simulink model "LPC_rec"  (Simulink 5.0)
settings: Solver=FixedStepDiscrete  SolverMode=SingleTasking  StartTime=0.0  StopTime=inf  RelTol=1e-3
PreLoadFcn:
  | load mtlb;
libraries: dspstat3 x2, dspbuff3 x2, dspsigops x2, dspsolvers x2, dsparch4 x2, dspsrcs4 x2
settings Model: RequirementInfo=9  CovMetricSettings=d  Creator=dshpak  LastModifiedBy=Miky  ExtModeTrigMode=oneshot  ExtModeArmWhenConnect=off  ExtModeAutoUpdateStatusClock=off  SaveTime=off  SaveOutput=off  SaveFormat=Structure  LimitDataPoints=off  IntegerOverflowMsg=none  BlockReductionOpt=off  BooleanDataType=off  RTWOptions="-aEnforceIntegerDowncast=1 -aExtMode=0 -aExtModeTesting=0 -aFoldNonRolledExpr=1 -aForceParamTrailComments=0 -aGenerateComments=1 -aGenerateReport=0 -aIgnoreCustomStorageClasses=1 -aIncDataTypeInIds=0 -aIncHierarchyInIds=0 -aInlineInvariantSignals=0 -aInlinedPrmAccess=\"Literals\" -aLocalBlockOutputs=1 -aLogVarNameModifier=\"rt_\" -aMaxRTWIdLen=31 -aPrefixModelToSubsysFcnNames=1 -aRTWVerbose=1 -aRollThreshold=5 -aShowEliminatedStatements=1"

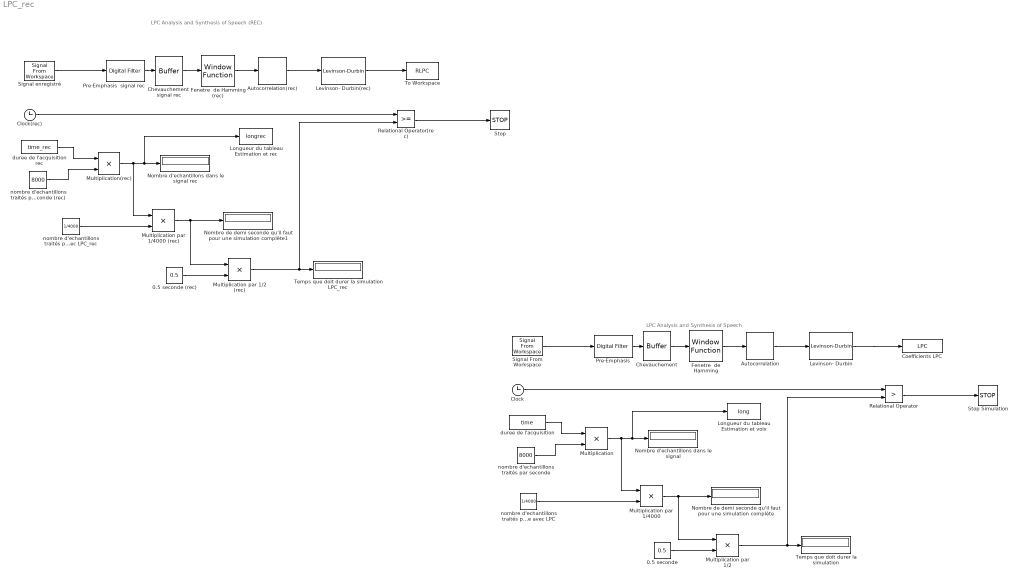
== system LPC_rec ==
  note: LPC Analysis and Synthesis of Speech
  note: LPC Analysis and Synthesis of Speech
      | (REC)
  0.5 seconde : Constant  Value=0.5
  0.5 seconde (rec) : Constant  Value=0.5
  Autocorrelation : dspstat3/Autocorrelation  AllPositiveLags=off  maxlag=12  bias=Biased  domain=Time
  Autocorrelation(rec) : dspstat3/Autocorrelation  AllPositiveLags=off  maxlag=12  bias=Biased  domain=Time
  Chevauchement : dspbuff3/Buffer  N=160  V=80  ic=0
  Chevauchement  signal rec : dspbuff3/Buffer  N=160  V=80  ic=0
  Clock : Clock
      settings: Decimation=10
  Clock(rec) : Clock
      settings: Decimation=10
  Coefficients LPC : ToWorkspace  VariableName=LPC  SampleTime=-1  SaveFormat=Array
  Fenetre  de Hamming : dspsigops/Window Function  winmode=Apply window to input  wintype=Hamming  N=64  Rs=50  beta=10  winsamp=Symmetric  UserWindow=hamming  OptParams=off  UserParams={1.0}  datatype=Double
  Fenetre  de Hamming (rec) : dspsigops/Window Function  winmode=Apply window to input  wintype=Hamming  N=64  Rs=50  beta=10  winsamp=Symmetric  UserWindow=hamming  OptParams=off  UserParams={1.0}  datatype=Double
  Levinson- Durbin : dspsolvers/Levinson-Durbin  coeffOutFcn=A  outP=off  zeroInpHandling=on
  Levinson- Durbin(rec) : dspsolvers/Levinson-Durbin  coeffOutFcn=A  outP=off  zeroInpHandling=on
  Longueur du tableau Estimation et rec : ToWorkspace  VariableName=longrec  SampleTime=-1  SaveFormat=StructureWithTime
      settings: MaxDataPoints=1
  Longueur du tableau Estimation et voix : ToWorkspace  VariableName=long  SampleTime=-1  SaveFormat=StructureWithTime
      settings: MaxDataPoints=1
  Multiplication : Product  Inputs=**  ShowAdditionalParam=on  OutDataTypeMode=single  OutScaling=2^-10
  Multiplication par 1/2 : Product  Inputs=**  ShowAdditionalParam=on  OutDataTypeMode=double  OutScaling=2^-10
  Multiplication par 1/2 (rec) : Product  Inputs=**  ShowAdditionalParam=on  OutDataTypeMode=double  OutScaling=2^-10
  Multiplication par 1/4000 : Product  Inputs=**  OutDataTypeMode=single  OutScaling=2^-10
  Multiplication par 1/4000 (rec) : Product  Inputs=**  OutDataTypeMode=single  OutScaling=2^-10
  Multiplication(rec) : Product  Inputs=**  ShowAdditionalParam=on  OutDataTypeMode=single  OutScaling=2^-10
  Nombre d'echantillons dans le signal : Display
  Nombre d'echantillons dans le signal rec : Display
  Nombre de demi seconde qu'il faut pour une simulation complète : Display
  Nombre de demi seconde qu'il faut pour une simulation complète1 : Display
  Pre-Emphasis : dsparch4/Digital Filter  TypePopup=FIR (all zeros)  IIRFiltStruct=Direct form II transposed  AllPoleFiltStruct=Direct form  FIRFiltStruct=Direct form  CoeffSource=Specify via dialog  NumCoeffs=[1 -.95]  DenCoeffs=[1 0.1]  BiQuadCoeffs=[1 0.3 0.4 1 0.1 0.2]  LatticeCoeffs=[0.2 0.4]  denIgnore=on  FiltPerSampPopup=One filter per frame  IC=0  ICnum=0  ICden=0
  Pre-Emphasis  signal rec : dsparch4/Digital Filter  TypePopup=FIR (all zeros)  IIRFiltStruct=Direct form II transposed  AllPoleFiltStruct=Direct form  FIRFiltStruct=Direct form  CoeffSource=Specify via dialog  NumCoeffs=[1 -.95]  DenCoeffs=[1 0.1]  BiQuadCoeffs=[1 0.3 0.4 1 0.1 0.2]  LatticeCoeffs=[0.2 0.4]  denIgnore=on  FiltPerSampPopup=One filter per frame  IC=0  ICnum=0  ICden=0
  Relational Operator : RelationalOperator  Operator=>
  Relational Operator(rec) : RelationalOperator
  Signal From Workspace : dspsrcs4/Signal From Workspace  X=voix  Ts=1/8000  nsamps=160  OutputAfterFinalValue=Setting to zero
  Signal enregistré : dspsrcs4/Signal From Workspace  X=rec  Ts=1/8000  nsamps=160  OutputAfterFinalValue=Setting to zero
  Stop : Stop
  Stop Simulation : Stop
  Temps que doit durer la simulation : Display
  Temps que doit durer la simulation LPC_rec : Display
  To Workspace : ToWorkspace  VariableName=RLPC  SampleTime=-1  SaveFormat=Array
  duree de l'acquisition : FromWorkspace  VariableName=time  SampleTime=0
  duree de l'acquisition rec : FromWorkspace  VariableName=time_rec  SampleTime=0
  nombre d'echantillons traités par 0.5 seconde avec LPC : Constant  Value=1/4000
  nombre d'echantillons traités par 0.5 seconde avec LPC_rec : Constant  Value=1/4000
  nombre d'echantillons traités par seconde : Constant  Value=8000  ShowAdditionalParam=on  OutDataTypeMode=double
  nombre d'echantillons traités par seconde (rec) : Constant  Value=8000  ShowAdditionalParam=on  OutDataTypeMode=double
  wires:
  Autocorrelation/1 -> Levinson- Durbin/1
  Fenetre  de Hamming/1 -> Autocorrelation/1
  Levinson- Durbin/1 -> Coefficients LPC/1
  Signal From Workspace/1 -> Pre-Emphasis/1
  Pre-Emphasis/1 -> Chevauchement/1
  Chevauchement/1 -> Fenetre  de Hamming/1
  Clock/1 -> Relational Operator/1
  Relational Operator/1 -> Stop Simulation/1
  nombre d'echantillons traités par seconde/1 -> Multiplication/2
  Multiplication/1 -> Multiplication par 1/4000/1, Nombre d'echantillons dans le signal/1, Longueur du tableau Estimation et voix/1
  Multiplication par 1/4000/1 -> Nombre de demi seconde qu'il faut pour une simulation complète/1, Multiplication par 1/2/1
  nombre d'echantillons traités par 0.5 seconde avec LPC/1 -> Multiplication par 1/4000/2
  0.5 seconde/1 -> Multiplication par 1/2/2
  Multiplication par 1/2/1 -> Temps que doit durer la simulation/1, Relational Operator/2
  duree de l'acquisition/1 -> Multiplication/1
  Autocorrelation(rec)/1 -> Levinson- Durbin(rec)/1
  Fenetre  de Hamming (rec)/1 -> Autocorrelation(rec)/1
  Signal enregistré/1 -> Pre-Emphasis  signal rec/1
  Pre-Emphasis  signal rec/1 -> Chevauchement  signal rec/1
  Chevauchement  signal rec/1 -> Fenetre  de Hamming (rec)/1
  Clock(rec)/1 -> Relational Operator(rec)/1
  Relational Operator(rec)/1 -> Stop/1
  nombre d'echantillons traités par seconde (rec)/1 -> Multiplication(rec)/2
  Multiplication(rec)/1 -> Multiplication par 1/4000 (rec)/1, Nombre d'echantillons dans le signal rec/1, Longueur du tableau Estimation et rec/1
  Multiplication par 1/4000 (rec)/1 -> Nombre de demi seconde qu'il faut pour une simulation complète1/1, Multiplication par 1/2 (rec)/1
  nombre d'echantillons traités par 0.5 seconde avec LPC_rec/1 -> Multiplication par 1/4000 (rec)/2
  0.5 seconde (rec)/1 -> Multiplication par 1/2 (rec)/2
  Multiplication par 1/2 (rec)/1 -> Temps que doit durer la simulation LPC_rec/1, Relational Operator(rec)/2
  duree de l'acquisition rec/1 -> Multiplication(rec)/1
  Levinson- Durbin(rec)/1 -> To Workspace/1
